simulink model "ICE"  (R2023a)
settings: Solver=VariableStepAuto  StartTime=0.0  StopTime=10.0  RelTol=1e-3
libraries: simulink x1
settings Model: Creator=Pedro  LastModifiedBy=Pedro

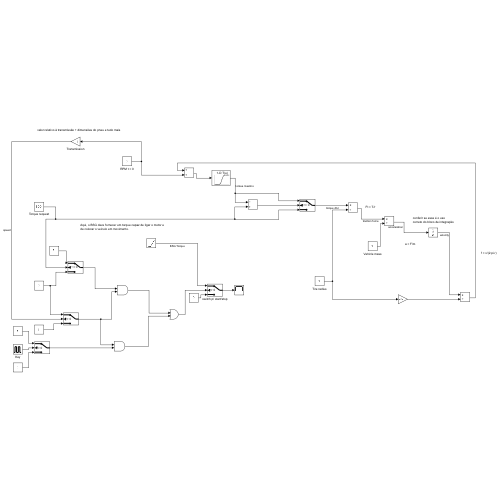
[thumbnail: Simulink's stored preview of the top-level diagram]
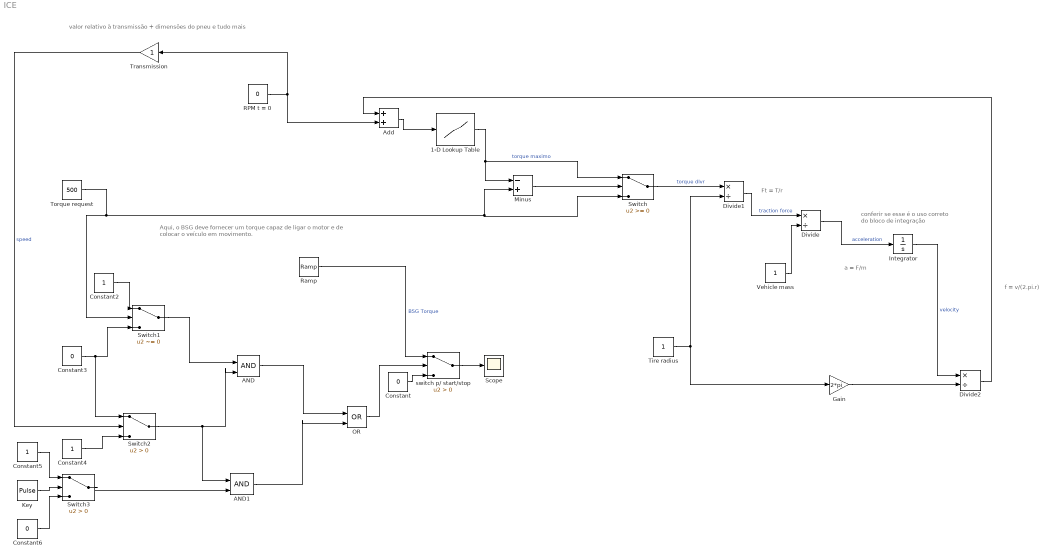
== system ICE ==
  note: a = F/m
  note: f = v/(2.pi.r)
  note: Ft = T/r
  note: conferir se esse é o uso
      | correto do bloco de integração
  note: valor relativo à transmissão + dimensões do pneu e tudo mais
  note: Aqui, o BSG deve fornecer um torque capaz de ligar o motor e
      | de colocar o veículo em movimento.
  1-D Lookup Table : Lookup_n-D  NumberOfTableDimensions=1  BreakpointsForDimension1=[-5:5]  Table=tanh([-5:5])  InternalRulePriority=Speed  RndMeth=Simplest
  AND : Logic  IconShape=distinctive  AllPortsSameDT=off  OutDataTypeStr=boolean
  AND1 : Logic  IconShape=distinctive  AllPortsSameDT=off  OutDataTypeStr=boolean
  Add : Sum
  Constant : Constant  Value=0
  Constant2 : Constant
  Constant3 : Constant  Value=0
  Constant4 : Constant
  Constant5 : Constant
  Constant6 : Constant  Value=0
  Divide : Product  Inputs=*/
  Divide1 : Product  Inputs=*/
  Divide2 : Product  Inputs=*/
  Gain : Gain  Gain=2*pi
  Integrator : Integrator
  Key : DiscretePulseGenerator  PulseType=Time based  Period=1  PulseWidth=5
  Minus : Sum  Inputs=-+
  OR : Logic  Operator=OR  IconShape=distinctive  AllPortsSameDT=off  OutDataTypeStr=boolean
  RPM t = 0 : Constant  Value=0
  Ramp : simulink/Sources/Ramp  slope=10  start=0  InitialOutput=0
  Scope : Scope
  Switch : Switch  SaturateOnIntegerOverflow=off  InputSameDT=off
  Switch1 : Switch  Criteria=u2 ~= 0  SaturateOnIntegerOverflow=off  InputSameDT=off
  Switch2 : Switch  Criteria=u2 > Threshold  SaturateOnIntegerOverflow=off  InputSameDT=off
  Switch3 : Switch  Criteria=u2 > Threshold  SaturateOnIntegerOverflow=off  InputSameDT=off
  Tire radius : Constant
  Torque request : Constant  Value=500
  Transmission : Gain
  Vehicle mass : Constant
  switch p/ start/stop : Switch  Criteria=u2 > Threshold  SaturateOnIntegerOverflow=off  InputSameDT=off
  wires:
  1-D Lookup Table/1 -> Switch/1, Minus/1  "torque maximo"
  Torque request/1 -> Switch1/2, Switch/3, Minus/2
  Minus/1 -> Switch/2
  Switch/1 -> Divide1/1  "torque dlvr"
  Transmission/1 -> Switch2/2  "speed"
  Switch1/1 -> AND/1
  Switch2/1 -> AND1/1, AND/2
  Ramp/1 -> switch p/ start/stop/1  "BSG Torque"
  Constant/1 -> switch p/ start/stop/3
  AND/1 -> OR/1
  AND1/1 -> OR/2
  OR/1 -> switch p/ start/stop/2
  Switch3/1 -> AND1/2
  Key/1 -> Switch3/2
  switch p/ start/stop/1 -> Scope/1
  Divide1/1 -> Divide/1  "traction force"
  Vehicle mass/1 -> Divide/2
  Tire radius/1 -> Divide1/2, Gain/1
  Divide/1 -> Integrator/1  "acceleration"
  Integrator/1 -> Divide2/1  "velocity"
  Gain/1 -> Divide2/2
  Add/1 -> 1-D Lookup Table/1
  RPM t = 0/1 -> Add/2, Transmission/1
  Divide2/1 -> Add/1
  Constant2/1 -> Switch1/1
  Constant3/1 -> Switch2/1, Switch1/3
  Constant4/1 -> Switch2/3
  Constant5/1 -> Switch3/1
  Constant6/1 -> Switch3/3
